simulink model "adrc_eso2"  (Simulink 7.5)
settings: Solver=ode45  StartTime=0.0  StopTime=10  RelTol=1e-3
undefined symbols (not defined in the file): a, b, wc, wo
settings Model: Creator=jasontatsumi  LastModifiedBy=jasontatsumi

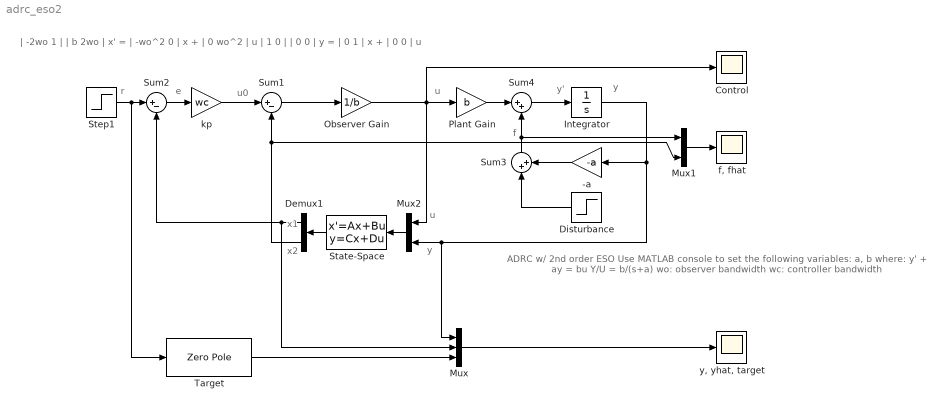
== system adrc_eso2 ==
  note: y
  note: y'
  note: f
  note: u
  note: u0
  note: y
  note: u
  note: x1
  note: x2
  note: ADRC w/ 2nd order ESO
      |
      | Use MATLAB console
      | to set the following
      | variables:
      |
      | a, b where:
      | y' + ay = bu
      | Y/U = b/(s+a)
      |
      | wo: observer bandwidth
      | wc: controller bandwidth
  note: | -2wo  1 |     | b 2wo  |
      | x' = | -wo^2 0 | x + | 0 wo^2 | u
      |
      |      | 1 0 |     | 0 0 |
      | y  = | 0 1 | x + | 0 0 | u
  note: e
  note: r
  -a : Gain  Gain=-a  ParameterDataType=fixdt(1, 16)  ParameterScaling=2^0  OutDataType=fixdt(1, 16)  OutScaling=2^0
  Control : Scope
      settings: TimeRange=10  YMin=0  YMax=1
  Demux1 : Demux  Outputs=2
  Disturbance : Step  Time=6  After=10  SampleTime=0
  Integrator : Integrator
  Mux : Mux  Inputs=3
  Mux1 : Mux  Inputs=2
  Mux2 : Mux  Inputs=2
  Observer Gain : Gain  Gain=1/b  ParameterDataType=fixdt(1, 16)  ParameterScaling=2^0  OutDataType=fixdt(1, 16)  OutScaling=2^0
  Plant Gain : Gain  Gain=b  ParameterDataType=fixdt(1, 16)  ParameterScaling=2^0  OutDataType=fixdt(1, 16)  OutScaling=2^0
  State-Space : StateSpace  A=[-2*wo 1;-wo^2 0]  B=[b 2*wo; 0 wo^2]  C=eye(2)  D=zeros(2,2)
  Step1 : Step  SampleTime=0
  Sum1 : Sum  Inputs=|+-  OutDataType=fixdt(1, 16)  OutScaling=2^0
  Sum2 : Sum  Inputs=|+-  OutDataType=fixdt(1, 16)  OutScaling=2^0
  Sum3 : Sum  Inputs=|++  OutDataType=fixdt(1, 16)  OutScaling=2^0
  Sum4 : Sum  Inputs=|++  OutDataType=fixdt(1, 16)  OutScaling=2^0
  Target : ZeroPole  Zeros=[]  Poles=[-wc]  Gain=[wc]
  "f, fhat" : Scope
      settings: TimeRange=10  YMin=0  YMax=1  SaveName=ScopeData2
  kp : Gain  Gain=wc  ParameterDataType=fixdt(1, 16)  ParameterScaling=2^0  OutDataType=fixdt(1, 16)  OutScaling=2^0
  "y, yhat, target" : Scope
      settings: TimeRange=10  YMin=0  YMax=1
  wires:
  Sum1/1 -> Observer Gain/1
  Mux2/1 -> State-Space/1
  State-Space/1 -> Demux1/1
  Integrator/1 -> -a/1, Mux2/2, Mux/1
  Sum2/1 -> kp/1
  Step1/1 -> Sum2/1, Target/1
  kp/1 -> Sum1/1
  Sum4/1 -> Integrator/1
  Observer Gain/1 -> Mux2/1, Plant Gain/1, Control/1
  Demux1/2 -> Sum1/2, Mux1/2
  Demux1/1 -> Sum2/2, Mux/2
  -a/1 -> Sum3/2
  Disturbance/1 -> Sum3/1
  Plant Gain/1 -> Sum4/1
  Sum3/1 -> Sum4/2, Mux1/1
  Mux/1 -> "y, yhat, target"/1
  Mux1/1 -> "f, fhat"/1
  Target/1 -> Mux/3
